simulink model "MCR2_Puzzlebot_Simulink_Example"  (R2024a)
settings: Solver=VariableStepAuto  StartTime=0.0  StopTime=90  RelTol=1e-3
undefined symbols (not defined in the file): Angular, Linear
libraries: robotlib x5, robotgazebolib x1, robotmobilelib x1, robotalgslib x1, robotcorelib x1
settings Model: Creator=mario  LastModifiedBy=mario

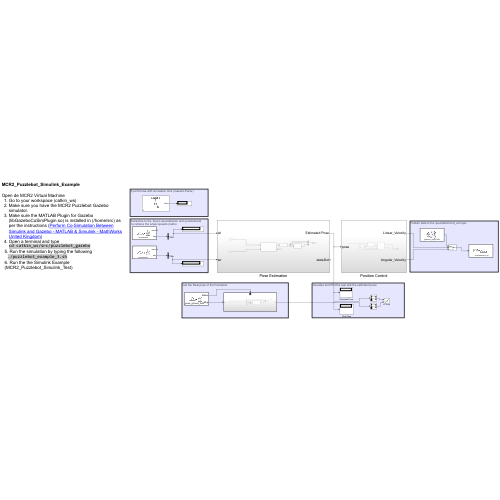
[thumbnail: Simulink's stored preview of the top-level diagram]
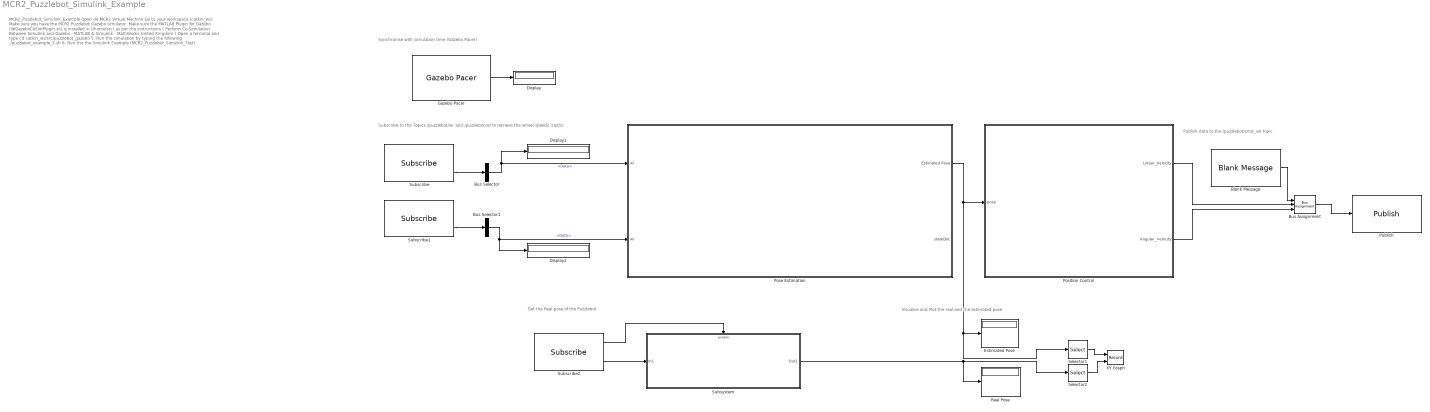
== system MCR2_Puzzlebot_Simulink_Example ==
  note: MCR2_Puzzlebot_Simulink_Example
      |
      | Open de MCR2 Virtual Machine
      | Go to your workspace (catkin_ws)
      | Make sure you have the MCR2 Puzzlebot Gazebo simulator.
      | Make sure the MATLAB Plugin for Gazebo (libGazeboCoSimPlugin.so) is installed in (/home/src) as per the instructions ( Perform Co-Simulation Between Simulink and Gazebo - MATLAB & Simulink - MathWorks United Kingdom )
      | Open a terminal and type
      | cd catkin_ws/src/puzzlebot_gazebo
      | 5. Run the simulation by typing the following
      | ./puzzlebot_example_3.sh
      | 6. Run the the Simulink Example (MCR2_Puzzlebot_Simulink_Test)
  note: Synchronise with simulation time (Gazebo Pacer)
  note: Publish data to the /puzzlebot/cmd_vel topic
  note: Visualise and Plot the real and the estimated pose
  note: Subscribe to the Topics /puzzlebot/wr and /puzzlebot/wl
      |  to retrieve the wheel speeds (rad/s)
  note: Get the Real pose of the Puzzlebot
  Blank Message : robotlib/Blank Message  messageClass=Message  entityType=geometry_msgs/Twist  messageType=geometry_msgs/Twist  SampleTime=-1  legacyBusStruct=off
  Bus Assignment : BusAssignment  AssignedSignals=Linear.X,Angular.Z
  Bus Selector : BusSelector  OutputSignals=Data
  Bus Selector1 : BusSelector  OutputSignals=Data
  Display : Display
  Display1 : Display
  Display2 : Display
  Estimated Pose : Display
  Gazebo Pacer : robotgazebolib/Gazebo Pacer  ResetBehavior=Reset Gazebo simulation time and scene  SampleTime=0.001
  Pose Estimation : Subsystem
  Position Control : Subsystem
  Publish : robotlib/Publish  topicSource=Select from ROS network  topic=/puzzlebot/cmd_vel  messageType=geometry_msgs/Twist  legacyBusStruct=off  messageQueueLength=1
  Real Pose : Display
  Selector1 : Selector  InputPortWidth=3  IndexOptions=Index vector (dialog)  Indices=[1 2]  OutputSizes=1
  Selector2 : Selector  InputPortWidth=3  IndexOptions=Index vector (dialog)  Indices=[1 2]  OutputSizes=1
  Subscribe : robotlib/Subscribe  topicSource=Select from ROS network  topic=/puzzlebot/wl  messageType=std_msgs/Float32  SampleTime=0.02  legacyBusStruct=off  messageQueueLength=1
  Subscribe1 : robotlib/Subscribe  topicSource=Select from ROS network  topic=/puzzlebot/wr  messageType=std_msgs/Float32  SampleTime=0.02  legacyBusStruct=off  messageQueueLength=1
  Subscribe2 : robotlib/Subscribe  topicSource=Select from ROS network  topic=/puzzlebot/base_pose_ground_truth  messageType=nav_msgs/Odometry  SampleTime=0.02  legacyBusStruct=off  messageQueueLength=1
  Subsystem : Subsystem
  XY Graph : Record  FileSettingsInternal="{\"entries\":[{\"content\":{\"excelSettings\":{\"content\":{},\"type\":\"Streamout.ExcelSettings\"}},\"type\":\"Streamout.FileSettingStorage\",\"uuid\":\"\"}],\"packageUris\":[\"http:\\/\\/schema.mathworks.com\\/mf0\\/streamout_blocks\\/R2020a\"],\"version\":\"1.0\"}"  Layout=[1 1]  SignalsInternal="{\"entries\":[{\"content\":{\"signals\":[{\"content\":{\"blockPath\":[],\"dimensions\":[2],\"domain\":\"\",\"hasChildren\":true,\"lineColor\":\"#4dbeee\",\"lineWidth\":2,\"port\":1,\"signalID\":1,\"signalName\":\"Mux3\"},\"type\":\"RecordBlkView.Signal\",\"uuid\":\"\"},{\"content\":{\"blockPath\":[],\"channel\":[1],\"dimensions\":[2],\"domain\":\"\",\"lineColor\":\"#a2142f\",\"lineWidth\":2,\"parentID\":1,\"plots\":[ 1 ],\"port\":1,\"signalID\":2,\"signalName\":\"Mux3\"},\"type\":\"RecordBlkView.Signal\",\"uuid\":\"\"},{\"content\":{\"blockPath\":[],\"channel\":[2],\"dimensions\":[2],\"domain\":\"\",\"lineColor\":\"#b746ff\",\"lineWidth\":2,\"parentID\":1,\"plots\":[ 1 ],\"port\":1,\"signalID\":3,\"signalName\":\"Mux3\"},\"type\":\"RecordBlkView.Signal\",\"uuid\":\"\"},{\"content\":{\"blockPath\":[],\"dimensions\":[2],\"domain\":\"\",\"hasChildren\":true,\"lineColor\":\"#139fff\",\"lineWidth\":2,\"port\":2,\"signalID\":4,\"signalName\":\"Mux4\"},\"type\":\"RecordBlkView.Signal\",\"uuid\":\"\"},{\"content\":{\"blockPath\":[],\"channel\":[1],\"dimensions\":[2],\"domain\":\"\",\"lineColor\":\"#ff6929\",\"lineWidth\":2,\"parentID\":4,\"plots\":[ 1 ],\"port\":2,\"signalID\":5,\"signalName\":\"Mux4\"},\"type\":\"RecordBlkView.Signal\",\"uuid\":\"\"},{\"content\":{\"blockPath\":[],\"channel\":[2],\"dimensions\":[2],\"domain\":\"\",\"lineColor\":\"#64d413\",\"lineWidth\":2,\"parentID\":4,\"plots\":[ 1 ],\"port\":2,\"signalID\":6,\"signalName\":\"Mux4\"},\"type\":\"RecordBlkView.Signal\",\"uuid\":\"\"}]},\"type\":\"RecordBlkView.InputSignals\",\"uuid\":\"\"}],\"packageUris\":[\"http:\\/\\/schema.mathworks.com\\/mf0\\/streamout_blocks\\/R2020a\"],\"version\":\"1.0\"}"  VisualizationBindings="{\"xyplotplugin\":{\"info\":[{\"series\":[{\"bindingParametersList\":[{\"parameter\":\"X-Axis\",\"signalID\":5,\"signalName\":\"Mux4(1)\"},{\"parameter\":\"Y-Axis\",\"signalID\":6,\"signalName\":\"Mux4(2)\"}],\"seriesID\":0},{\"bindingParametersList\":[{\"parameter\":\"X-Axis\",\"signalID\":2,\"signalName\":\"Mux3(1)\"},{\"parameter\":\"Y-Axis\",\"signalID\":3,\"signalName\":\"Mux3(2)\"}],\"seriesID\":1}],\"subplotID\":1}]}}"  CompatibilityTag=XY
  wires:
  Gazebo Pacer/1 -> Display/1
  Subscribe/2 -> Bus Selector/1
  Bus Selector/1 -> Display1/1, Pose Estimation/1(wl)  "<Data>"
  Blank Message/1 -> Bus Assignment/1
  Bus Assignment/1 -> Publish/1
  Subscribe1/2 -> Bus Selector1/1
  Bus Selector1/1 -> Display2/1, Pose Estimation/2(wr)  "<Data>"
  Selector2/1 -> XY Graph/2
  Selector1/1 -> XY Graph/1
  Pose Estimation/1(Estimated Pose) -> Estimated Pose/1, Selector1/1, Position Control/1(pose)
  Subsystem/1(Out1) -> Real Pose/1, Selector2/1
  Subscribe2/2 -> Subsystem/1(In1)
  Subscribe2/1 -> Subsystem/Enable
  Position Control/1(Linear_Velocity) -> Bus Assignment/2
  Position Control/2(Angular_Velocity) -> Bus Assignment/3

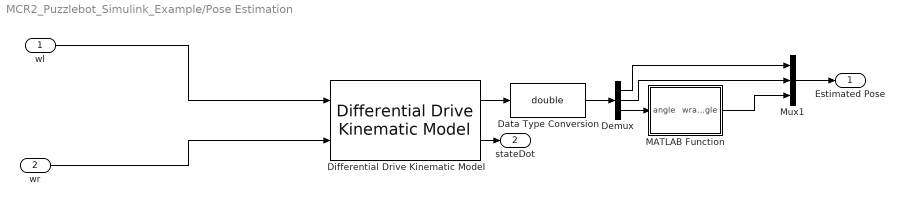
== system MCR2_Puzzlebot_Simulink_Example/Pose Estimation ==
  wl : Inport
  wr : Inport  Port=2
  Data Type Conversion : DataTypeConversion  OutDataTypeStr=double  SaturateOnIntegerOverflow=off  RndMeth=Floor
  Demux : Demux  Outputs=3
  Differential Drive Kinematic Model : robotmobilelib/Differential Drive Kinematic Model  VehicleInputs=Wheel Speeds  WheelRadius=0.05  WheelSpeedRange=[-Inf Inf]  TrackWidth=0.19  InitialState=[-2; -2; 0]  SimulateUsing=Code generation
  MATLAB Function : MATLAB Function  TreatAsAtomicUnit=on
  Mux1 : Mux  Inputs=3
  Estimated Pose : Outport
  stateDot : Outport  Port=2
  wires:
  Demux/1 -> Mux1/1
  MATLAB Function/1(wrapped_angle) -> Mux1/3
  wr/1 -> Differential Drive Kinematic Model/2
  wl/1 -> Differential Drive Kinematic Model/1
  Differential Drive Kinematic Model/1 -> Data Type Conversion/1
  Demux/3 -> MATLAB Function/1(angle)
  Demux/2 -> Mux1/2
  Data Type Conversion/1 -> Demux/1
  Mux1/1 -> Estimated Pose/1
  Differential Drive Kinematic Model/2 -> stateDot/1

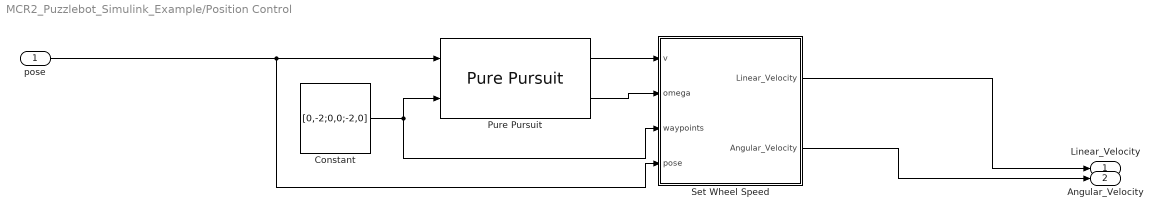
== system MCR2_Puzzlebot_Simulink_Example/Position Control ==
  pose : Inport
  Constant : Constant  Value=[0,-2;0,0;-2,0]  VectorParams1D=off  OutDataTypeStr=double
  Pure Pursuit : robotalgslib/Pure Pursuit  DesiredLinearVelocityPort=off  DesiredLinearVelocity=.5  MaxAngularVelocity=0.5  LookaheadDistancePort=off  LookaheadDistance=0.5  TargetDirPort=off  SimulateUsing=Code generation
      settings: LibrarySourceBlock=robotmobilelib/Pure Pursuit
  Set Wheel Speed : MATLAB Function  TreatAsAtomicUnit=on
  Linear_Velocity : Outport
  Angular_Velocity : Outport  Port=2
  wires:
  Set Wheel Speed/2(Angular_Velocity) -> Angular_Velocity/1
  Pure Pursuit/1 -> Set Wheel Speed/1(v)
  Set Wheel Speed/1(Linear_Velocity) -> Linear_Velocity/1
  Constant/1 -> Pure Pursuit/2, Set Wheel Speed/3(waypoints)
  pose/1 -> Pure Pursuit/1, Set Wheel Speed/4(pose)
  Pure Pursuit/2 -> Set Wheel Speed/2(omega)

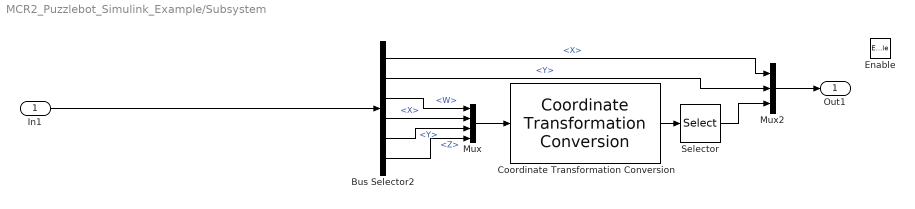
== system MCR2_Puzzlebot_Simulink_Example/Subsystem ==
  In1 : Inport
  Enable : EnablePort
  Bus Selector2 : BusSelector  OutputSignals=Pose.Pose.Position.X,Pose.Pose.Position.Y,Pose.Pose.Orientation.W,Pose.Pose.Orientation.X,Pose.Pose.Orientation.Y,Pose.Pose.Orientation.Z
  Coordinate Transformation Conversion : robotcorelib/Coordinate Transformation Conversion  InputRepresentation=Quaternion  InputEulerSequence=ZYX  ShowTrVecInputPort=on  OutputRepresentation=Euler Angles  OutputEulerSequence=ZYX  ShowTrVecOutputPort=on  SimulateUsing=Interpreted execution
      settings: LibrarySourceBlock=roslib/Utilities/Coordinate Transformation Conversion
  Mux : Mux
  Mux2 : Mux  Inputs=3
  Selector : Selector  InputPortWidth=3  IndexOptions=Index vector (dialog)  Indices=1  OutputSizes=1
  Out1 : Outport
  wires:
  Bus Selector2/4 -> Mux/2  "<X>"
  Bus Selector2/1 -> Mux2/1  "<X>"
  Selector/1 -> Mux2/3
  Bus Selector2/5 -> Mux/3  "<Y>"
  Bus Selector2/3 -> Mux/1  "<W>"
  Bus Selector2/6 -> Mux/4  "<Z>"
  Mux/1 -> Coordinate Transformation Conversion/1
  Bus Selector2/2 -> Mux2/2  "<Y>"
  Mux2/1 -> Out1/1
  Coordinate Transformation Conversion/1 -> Selector/1
  In1/1 -> Bus Selector2/1

== matlab function MCR2_Puzzlebot_Simulink_Example/Position Control/Set Wheel Speed ==
  data: v input; omega input; waypoints input; pose input; Linear_Velocity output; Angular_Velocity output
function [Linear_Velocity, Angular_Velocity] = RobotSpeed(v, omega, waypoints, pose)

% Path constants
stopThreshold = 0.1;
slowThreshold = 0.3;

% Slow the robot down when it's near the threshold
distanceToEndpoint = norm(waypoints(end, :) - pose(1:2)');
if (distanceToEndpoint < slowThreshold)
    v = distanceToEndpoint/slowThreshold*v;
    omega = distanceToEndpoint/slowThreshold*omega;
    
    % Stop the robot if it's inside the target threshold
    if distanceToEndpoint < stopThreshold
        v = 0;
        omega = 0;
    end
end

% Convert velocity and heading angular velocity to wheel speeds
Linear_Velocity = v;
Angular_Velocity = omega;

end

== matlab function MCR2_Puzzlebot_Simulink_Example/Pose Estimation/MATLAB Function ==
  data: angle input; wrapped_angle output
function wrapped_angle = wrap2Pi(angle)

wrapped_angle = wrapToPi(angle);
